simulink model "admire_sim_wal"  (Simulink 3.00)
settings: Solver=ode4  SolverMode=SingleTasking  StartTime=0.0  StopTime=7.5  FixedStep=0.01  RelTol=1e-3  AbsTol=1e-6
values from neighbouring files (symbols this model uses):
  x0 = [ max(eyp,zeros(n,1));max(-eyp,zeros(n,1));zeros(2*m,1)]    [LPwrap.m]
undefined symbols (not defined in the file or in its folder): dalpha_err, dalt_err, dbeta_err, dCl_beta, dCl_dai, dCl_day, dCl_dr, dCl_p, dCl_r, dCm_alpha, dCm_dei, dCm_dey, dCm_dne, dCm_q, dCn_beta, dCn_dna, dCn_dr, dCn_p, dCn_r, dCn_zero, ddc_bw, ddc_rate, ddei_bw, ddei_rate, ddey_bw, ddey_rate, ddle_bw, ddle_rate, ddr_bw, ddr_rate, dIxx, dIxz, dIyy, dIzz, dmass, dVt_err, dxcg, dycg, dzcg, rlimit_c, rlimit_ie, rlimit_le, rlimit_oe, rlimit_r, u0corr, u0fcs, u0new, x0diff, y0bare
libraries: simulink_extras x27, simulink3 x22
(part 1 of 2)
settings Model: RTWOptions="-aLogVarNameModifier=\"rt_\" -aExtMode=0 -aRollThreshold=5 -aShowEliminatedStatements=1 -aRTWVerbose=1 -aInlineInvariantSignals=1 -aLocalBlockOutputs=1 -aInlineParameters=0"  RTWTemplateMakefile=grt_adm5p3.tmf  LastModifiedBy=hkg  ModifiedComment=nnt -- Mon Jun 05 13:08:11 2000 -- Version 3.42
settings Model: ModifiedHistory=|
  | nnt -- Mon Jun 05 13:08:11 2000 -- Version 3.42
  | 
  | 
  | nnt -- Mon Jun 05 11:01:33 2000 -- Version 3.41
  | 
  | 
  | nnt -- Mon Jun 05 10:57:40 2000 -- Version 3.40
  | 
  | 
  | nnt -- Mon Jun 05 10:56:46 2000 -- Version 3.39
  | 
  | 
  | hkg -- Thu Apr 13 16:38:30 2000 -- Version 3.38
  | Bug fix: all rate limiters were set with the canard parameters, now they get individual settings..
  | 
  | hkg -- Thu Apr 13 10:24:31 2000 -- Version 3.37
  | Inserted 3.0 version number in Level 1, changed month to April.
  | 
  | hkg -- Tue Apr 11 10:36:55 2000 -- Version 3.36
  | dtz re-connected
  | 
  | hkg -- Tue Apr 11 10:28:52 2000 -- Version 3.35
  | Changed the roll force saturation to +-80 N
  | 
  | hkg -- Tue Apr 11 09:23:02 2000 -- Version 3.34
  | All signal generators on Level 1 are now set to sine wave
  | 
  | hkg -- Mon Apr 10 15:03:16 2000 -- Version 3.33
  | New names for the RL_choice blocks
  | 
  | fosimadmin -- Mon Apr 10 13:44:14 2000 -- Version 3.32
  | Hkg actually. Nothing special
  | 
  | hkg -- Fri Apr 07 14:32:16 2000 -- Version 3.31
  | A few corrections to the names
  | 
  | hkg -- Fri Apr 07 14:16:55 2000 -- Version 3.30
  | Added unique names inside Saab and DASA rate limiters for left elevons, rudder and
  | leading-edge flaps.
  | hkg -- Fri Apr 07 14:04:35 2000 -- Version 3.29
  | Added unique names inside SAAB and DASA rate limiters for canard and right outer and
  | inner elevons.
  | hkg -- Thu Apr 06 17:23:24 2000 -- Version 3.28
  | Inserted unique names for rate limiters and multiport switches in the rate limiter selection blocks.
  | hkg -- Thu Apr 06 16:09:22 2000 -- Version 3.27
  | Disconnected dtz again. Chosen grt_adm5p3.tmf as template makefile. Code generation seems to work.
  | hyd -- Tue Mar 28 15:20:39 2000 -- Version 3.26
  | hyd -- Tue Mar 28 14:28:32 2000 -- Version 3.25
  | hyd -- Tue Mar 28 11:30:24 2000 -- Version 3.24
  | hyd -- Mon Mar 27 15:22:27 2000 -- Version 3.23
  | hyd -- Mon Mar 27 13:42:12 2000 -- Version 3.22
  | hyd -- Mon Mar 27 10:51:54 2000 -- Version 3.21
  | hyd -- Fri Mar 24 13:18:05 2000 -- Version 3.20
  | hyd -- Fri Mar 24 12:50:02 2000 -- Version 3.19
  | hyd -- Fri Mar 24 11:54:23 2000 -- Version 3.18
  | hyd -- Thu Mar 23 15:20:42 2000 -- Version 3.17
  | hyd -- Thu Mar 23 15:17:54 2000 -- Version 3.16
  | hyd -- Wed Mar 22 09:38:49 2000 -- Version 3.15
  | hyd -- Tue Mar 21 14:06:08 2000 -- Version 3.14
  | hyd -- Mon Mar 20 14:42:54 2000 -- Version 3.13
  | hyd -- Wed Mar 15 13:37:48 2000 -- Version 3.12
  | hyd -- Wed Mar 15 12:35:54 2000 -- Version 3.11
  | jnr -- Tue Mar 14 16:36:26 2000 -- Version 3.10
  | jnr -- Tue Mar 14 14:13:39 2000 -- Version 3.9
  | jnr -- Tue Mar 14 14:13:23 2000 -- Version 3.8
  | jnr -- Tue Mar 14 10:09:15 2000 -- Version 3.7
  | jnr -- Tue Mar 14 09:37:34 2000 -- Version 3.6
  | jnr -- Tue Mar 14 09:30:20 2000 -- Version 3.5
  | Add:
  | *proper stick gradients.
  | *correct gains for nz-control according to Åke Hydén.
  | *what transition region between q-control and nz-control is proper??
  | fll -- Fri Mar 03 09:53:48 2000 -- Version 3.4
  | changed name of "dtx" to "dty" (horizontal nozzle deflection)
  | fll -- Thu Mar 02 12:51:23 2000 -- Version 3.3
  | Reducesed the number of integrators to one in the longitudinal controller.
  | fll -- Thu Mar 02 12:30:52 2000 -- Version 3.2
  | Moved the blending function in the Nz and q controller.
  | fll -- Thu Mar 02 10:50:25 2000 -- Version 3.1
  | Changed input blocks to "Signal generator"
  | fll -- Thu Mar 02 10:50:25 2000 -- Version 3.0
  | Version 3.0 is modified according to comments from users

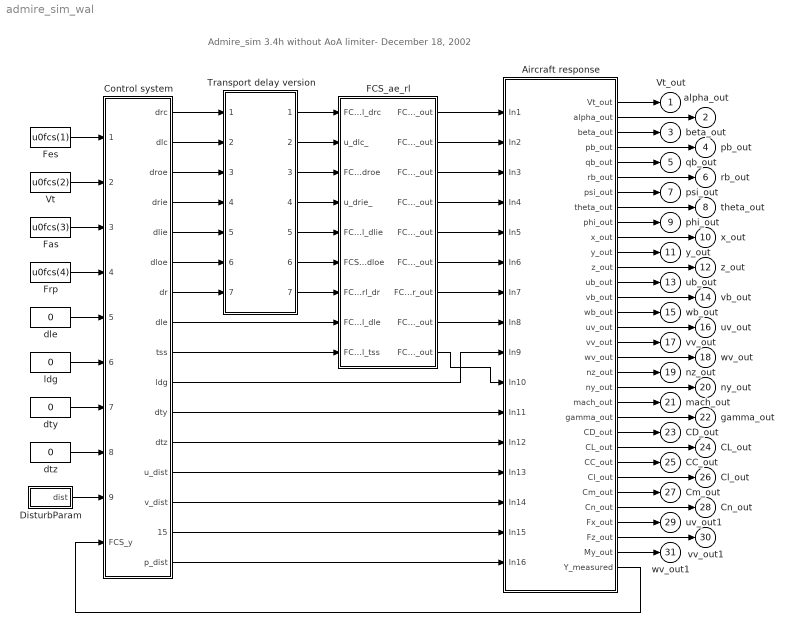
== system admire_sim_wal ==
  note: Admire_sim 3.4h without AoA limiter- December 18, 2002
  Aircraft response : Subsystem
      mask Display: disp('Aircraft\nResponse')
  Control system : Subsystem
      mask Display: disp('Control\nSystem')
  DisturbParam : Subsystem
  FCS_ae_rl : Subsystem
      mask Display: disp('Saturators\nRatelimiters\nand\nActuators')
  Fas : Constant  Value=u0fcs(3)
  Fes : Constant  Value=u0fcs(1)
  Frp : Constant  Value=u0fcs(4)
  Transport delay version : Subsystem
      mask Display: disp('Total\nComputer\nDelay\n\nTransport\ndelay\nversion')
  Vt : Constant  Value=u0fcs(2)
  dle : Constant  Value=0
  dty : Constant  Value=0
  dtz : Constant  Value=0
  ldg : Constant  Value=0
  Vt_out : Outport  Port=1  InitialOutput=0
  alpha_out : Outport  Port=2  InitialOutput=0
  beta_out : Outport  Port=3  InitialOutput=0
  pb_out : Outport  Port=4  InitialOutput=0
  qb_out : Outport  Port=5  InitialOutput=0
  rb_out : Outport  Port=6  InitialOutput=0
  psi_out : Outport  Port=7  InitialOutput=0
  theta_out : Outport  Port=8  InitialOutput=0
  phi_out : Outport  Port=9  InitialOutput=0
  x_out : Outport  Port=10  InitialOutput=0
  y_out : Outport  Port=11  InitialOutput=0
  z_out : Outport  Port=12  InitialOutput=0
  ub_out : Outport  Port=13  InitialOutput=0
  vb_out : Outport  Port=14  InitialOutput=0
  wb_out : Outport  Port=15  InitialOutput=0
  uv_out : Outport  Port=16  InitialOutput=0
  vv_out : Outport  Port=17  InitialOutput=0
  wv_out : Outport  Port=18  InitialOutput=0
  nz_out : Outport  Port=19  InitialOutput=0
  ny_out : Outport  Port=20  InitialOutput=0
  mach_out : Outport  Port=21  InitialOutput=0
  gamma_out : Outport  Port=22  InitialOutput=0
  CD_out : Outport  Port=23  InitialOutput=0
  CL_out : Outport  Port=24  InitialOutput=0
  CC_out : Outport  Port=25  InitialOutput=0
  Cl_out : Outport  Port=26  InitialOutput=0
  Cm_out : Outport  Port=27  InitialOutput=0
  Cn_out : Outport  Port=28  InitialOutput=0
  uv_out1 : Outport  Port=29  InitialOutput=0
  vv_out1 : Outport  Port=30  InitialOutput=0
  wv_out1 : Outport  Port=31  InitialOutput=0
  wires:
  Aircraft response/1(Vt_out) -> Vt_out/1
  Aircraft response/3(beta_out) -> beta_out/1
  Aircraft response/5(qb_out) -> qb_out/1
  Aircraft response/7(psi_out) -> psi_out/1
  Aircraft response/9(phi_out) -> phi_out/1
  Aircraft response/11(y_out) -> y_out/1
  Aircraft response/13(ub_out) -> ub_out/1
  Aircraft response/15(wb_out) -> wb_out/1
  Aircraft response/19(nz_out) -> nz_out/1
  FCS_ae_rl/8(FCS_ae_rl_dle_out) -> Aircraft response/8(In8)
  FCS_ae_rl/7(FCS_ae_rl_dr_out) -> Aircraft response/7(In7)
  FCS_ae_rl/6(FCS_ae_rl_dloe_out) -> Aircraft response/6(In6)
  FCS_ae_rl/5(FCS_ae_rl_dlie_out) -> Aircraft response/5(In5)
  FCS_ae_rl/4(FCS_ae_rl_drie_out) -> Aircraft response/4(In4)
  FCS_ae_rl/3(FCS_ae_rl_droe_out) -> Aircraft response/3(In3)
  FCS_ae_rl/2(FCS_ae_rl_dlc_out) -> Aircraft response/2(In2)
  FCS_ae_rl/1(FCS_ae_rl_drc_out) -> Aircraft response/1(In1)
  FCS_ae_rl/9(FCS_ae_rl_tss_out) -> Aircraft response/10(In10)
  Transport delay version/1(FCS_ae_rl_del_drc_delayed) -> FCS_ae_rl/1(FCS_ae_rl_drc)
  Transport delay version/2(FCS_ae_rl_del_dlc_delayed) -> FCS_ae_rl/2(u_dlc_)
  Transport delay version/3(FCS_ae_rl_del_droe_delayed) -> FCS_ae_rl/3(FCS_ae_rl_droe)
  Transport delay version/4(FCS_ae_rl_del_drie_delayed) -> FCS_ae_rl/4(u_drie_)
  Transport delay version/5(FCS_ae_rl_del_dlie_delayed) -> FCS_ae_rl/5(FCS_ae_rl_dlie)
  Transport delay version/6(FCS_ae_rl_del_dloe_delayed) -> FCS_ae_rl/6(FCS_ae_rl_dloe)
  Transport delay version/7(FCS_ae_rl_del_dr_delayed) -> FCS_ae_rl/7(FCS_ae_rl_dr)
  Aircraft response/17(vv_out) -> vv_out/1
  Aircraft response/21(mach_out) -> mach_out/1
  Aircraft response/23(CD_out) -> CD_out/1
  Aircraft response/25(CC_out) -> CC_out/1
  Aircraft response/27(Cm_out) -> Cm_out/1
  Aircraft response/29(Fx_out) -> uv_out1/1
  Aircraft response/31(My_out) -> wv_out1/1
  Aircraft response/2(alpha_out) -> alpha_out/1
  Aircraft response/22(gamma_out) -> gamma_out/1
  Aircraft response/4(pb_out) -> pb_out/1
  Aircraft response/6(rb_out) -> rb_out/1
  Aircraft response/8(theta_out) -> theta_out/1
  Aircraft response/10(x_out) -> x_out/1
  Aircraft response/14(vb_out) -> vb_out/1
  Aircraft response/16(uv_out) -> uv_out/1
  Aircraft response/18(wv_out) -> wv_out/1
  Aircraft response/20(ny_out) -> ny_out/1
  Aircraft response/12(z_out) -> z_out/1
  Aircraft response/24(CL_out) -> CL_out/1
  Aircraft response/26(Cl_out) -> Cl_out/1
  Aircraft response/28(Cn_out) -> Cn_out/1
  Aircraft response/30(Fz_out) -> vv_out1/1
  Control system/1(drc) -> Transport delay version/1(FCS_ae_rl_del_drc)
  Control system/2(dlc) -> Transport delay version/2(FCS_ae_rl_del_dlc)
  Control system/3(droe) -> Transport delay version/3(FCS_ae_rl_del_droe)
  Control system/4(drie) -> Transport delay version/4(FCS_ae_rl_del_drie)
  Control system/5(dlie) -> Transport delay version/5(FCS_ae_rl_del_dlie)
  Control system/6(dloe) -> Transport delay version/6(FCS_ae_rl_del_dloe)
  Control system/7(dr) -> Transport delay version/7(FCS_ae_rl_del_dr)
  Control system/8(dle) -> FCS_ae_rl/8(FCS_ae_rl_dle)
  Control system/9(tss) -> FCS_ae_rl/9(FCS_ae_rl_tss)
  Control system/10(ldg) -> Aircraft response/9(In9)
  Control system/11(dty) -> Aircraft response/11(In11)
  Control system/13(u_dist) -> Aircraft response/13(In13)
  Control system/14(v_dist) -> Aircraft response/14(In14)
  Control system/15(w_dist) -> Aircraft response/15(In15)
  Control system/16(p_dist) -> Aircraft response/16(In16)
  DisturbParam/1(dist) -> Control system/9(FCS_dist)
  dtz/1 -> Control system/8(FCS_dtz)
  dty/1 -> Control system/7(FCS_dty)
  ldg/1 -> Control system/6(FCS_ldg)
  dle/1 -> Control system/5(FCS_dle)
  Frp/1 -> Control system/4(FCS_Frp)
  Aircraft response/32(Y_measured) -> Control system/10(FCS_y)
  Control system/12(dtz) -> Aircraft response/12(In12)
  Fas/1 -> Control system/3(FCS_Fas)
  Vt/1 -> Control system/2(FCS_Vt)
  Fes/1 -> Control system/1(FCS_Fes)

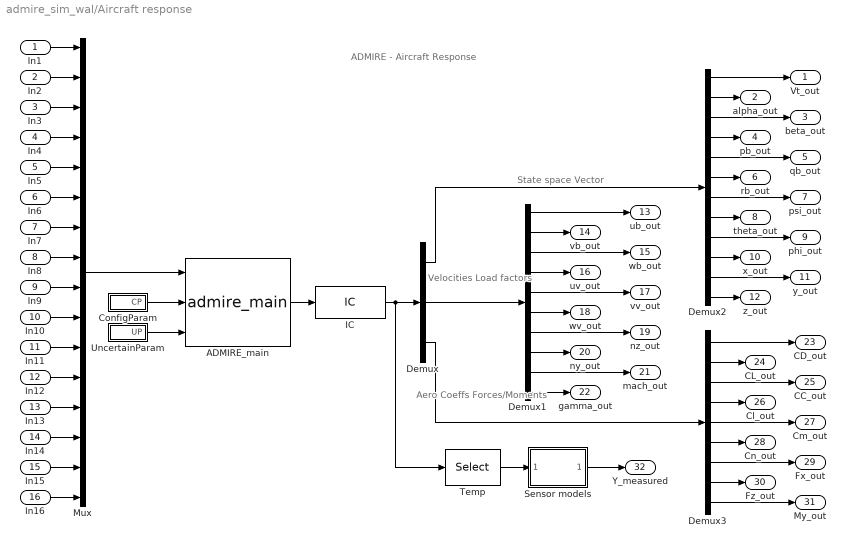
== system admire_sim_wal/Aircraft response ==
  note: State space Vector
  note: Velocities
      | Load factors
  note: Aero Coeffs
      | Forces/Moments
  note: ADMIRE - Aircraft Response
  In1 : Inport  Port=1  PortWidth=-1  SampleTime=-1  DataType=auto
      settings: SignalType=auto
  In2 : Inport  Port=2  PortWidth=-1  SampleTime=-1  DataType=auto
      settings: SignalType=auto
  In3 : Inport  Port=3  PortWidth=-1  SampleTime=-1  DataType=auto
      settings: SignalType=auto
  In4 : Inport  Port=4  PortWidth=-1  SampleTime=-1  DataType=auto
      settings: SignalType=auto
  In5 : Inport  Port=5  PortWidth=-1  SampleTime=-1  DataType=auto
      settings: SignalType=auto
  In6 : Inport  Port=6  PortWidth=-1  SampleTime=-1  DataType=auto
      settings: SignalType=auto
  In7 : Inport  Port=7  PortWidth=-1  SampleTime=-1  DataType=auto
      settings: SignalType=auto
  In8 : Inport  Port=8  PortWidth=-1  SampleTime=-1  DataType=auto
      settings: SignalType=auto
  In9 : Inport  Port=9  PortWidth=-1  SampleTime=-1  DataType=auto
      settings: SignalType=auto
  In10 : Inport  Port=10  PortWidth=-1  SampleTime=-1  DataType=auto
      settings: SignalType=auto
  In11 : Inport  Port=11  PortWidth=-1  SampleTime=-1  DataType=auto
      settings: SignalType=auto
  In12 : Inport  Port=12  PortWidth=-1  SampleTime=-1  DataType=auto
      settings: SignalType=auto
  In13 : Inport  Port=13  PortWidth=-1  SampleTime=-1  DataType=auto
      settings: SignalType=auto
  In14 : Inport  Port=14  PortWidth=-1  SampleTime=-1  DataType=auto
      settings: SignalType=auto
  In15 : Inport  Port=15  PortWidth=-1  SampleTime=-1  DataType=auto
      settings: SignalType=auto
  In16 : Inport  Port=16  PortWidth=-1  SampleTime=-1  DataType=auto
      settings: SignalType=auto
  ADMIRE_main : S-Function  FunctionName=admire_main  Parameters=x0bare dx0bare  PortCounts=[]  SFunctionModules=''
      mask Type: ADMIRE C-code block
      mask Description:
      | Main block describing the ADMIRE.
      | To use HELP, start any Internet browser.
      mask Help:
      | The aircraft it self is a C-code file that calculates the dynamics of the structure and the air surrounding it.<br>
      | The simulation requires an initial vector of values called x0 containing the following variables.<br><br>
      | 
      | Vt_init     --     initial airspeed.                        [m/s]<br>
      | alpha_init --    initial angle of attack.             [rad]<br>
      | beta_init    --   initial angle of sideslip.            [rad]<br>
      | pb_init     --     initial roll angular rate.             [rad/s]<br>
      | qb_init     --     initial pitch angular rate.          [rad/s]<br>
      | rb_init       --    initial yaw angular rate.           [rad/s]<br>
      | psi_init      --    initial euler angles (azimuth)    [rad]<br>
      | theta_init   --   initial (elevation)                      [rad]<br>
      | phi_init      --   initial (bank)                             [rad]<br>
      | xv_init      --    initial x position in Fv                [m]<br>
      | yv_init        --  initial y                                     [m]<br>
      | zv_init       --   initial z                                     [m]<br>
      mask Display:
      | plot([18 12 3 2 2 8 11],[7 4 1 1 2 8 11])
      | plot([13 11 13 15 15 13],[12 11 16 17 13 12])
      | plot([15 17 20 23 30 17],[13 14 24 25 20 14])
      | plot([30 38 40 38 30],[19 31 32 22 19])
      | plot([38.5 41 36 22 41 43 36],[23 21 16 10 8 10 16])
      | plot([15 19 25 24 15],[7 9 9 8 7])
      | plot([8 11 13 14 9 8],[8 11 12 10 7 8])
      | plot([21 23],[9 10])
      | plot([30 31],[20 20.5])
  ConfigParam : Subsystem
  Demux : Demux  Outputs=[12 10 9]
  Demux1 : Demux  Outputs=10
  Demux2 : Demux  Outputs=12
  Demux3 : Demux  Outputs=9
  IC : InitialCondition  Value=y0bare(1:31)
  Mux : Mux  Inputs=16
      settings: DisplayOption=none
  Sensor models : Subsystem
      mask Display: disp('Sensors')
  Temp : Selector  Elements=[1:28]  InputPortWidth=31
  UncertainParam : Subsystem
      mask Display: plot([0 10 5 0],[0 0 8.6603 0])
  Vt_out : Outport  Port=1
  alpha_out : Outport  Port=2
  beta_out : Outport  Port=3
  pb_out : Outport  Port=4
  qb_out : Outport  Port=5
  rb_out : Outport  Port=6
  psi_out : Outport  Port=7
  theta_out : Outport  Port=8
  phi_out : Outport  Port=9
  x_out : Outport  Port=10
  y_out : Outport  Port=11
  z_out : Outport  Port=12
  ub_out : Outport  Port=13
  vb_out : Outport  Port=14
  wb_out : Outport  Port=15
  uv_out : Outport  Port=16
  vv_out : Outport  Port=17
  wv_out : Outport  Port=18
  nz_out : Outport  Port=19
  ny_out : Outport  Port=20
  mach_out : Outport  Port=21
  gamma_out : Outport  Port=22
  CD_out : Outport  Port=23
  CL_out : Outport  Port=24
  CC_out : Outport  Port=25
  Cl_out : Outport  Port=26
  Cm_out : Outport  Port=27
  Cn_out : Outport  Port=28
  Fx_out : Outport  Port=29
  Fz_out : Outport  Port=30
  My_out : Outport  Port=31
  Y_measured : Outport  Port=32
  wires:
  Mux/1 -> ADMIRE_main/1
  In15/1 -> Mux/15
  In16/1 -> Mux/16
  In1/1 -> Mux/1
  In2/1 -> Mux/2
  In3/1 -> Mux/3
  In4/1 -> Mux/4
  In5/1 -> Mux/5
  In6/1 -> Mux/6
  In7/1 -> Mux/7
  In8/1 -> Mux/8
  In9/1 -> Mux/9
  In10/1 -> Mux/10
  In11/1 -> Mux/11
  In12/1 -> Mux/12
  In13/1 -> Mux/13
  In14/1 -> Mux/14
  Demux/2 -> Demux1/1
  Demux/1 -> Demux2/1
  Demux/3 -> Demux3/1
  Demux3/2 -> CL_out/1
  Demux3/4 -> Cl_out/1
  Demux3/6 -> Cn_out/1
  Demux3/8 -> Fz_out/1
  Demux3/1 -> CD_out/1
  Demux3/3 -> CC_out/1
  Demux3/5 -> Cm_out/1
  Demux3/7 -> Fx_out/1
  Demux3/9 -> My_out/1
  Demux2/2 -> alpha_out/1
  Demux2/4 -> pb_out/1
  Demux2/6 -> rb_out/1
  Demux2/8 -> theta_out/1
  Demux2/10 -> x_out/1
  Demux2/12 -> z_out/1
  Demux2/1 -> Vt_out/1
  Demux2/3 -> beta_out/1
  Demux2/5 -> qb_out/1
  Demux2/7 -> psi_out/1
  Demux2/9 -> phi_out/1
  Demux2/11 -> y_out/1
  Demux1/2 -> vb_out/1
  Demux1/4 -> uv_out/1
  Demux1/6 -> wv_out/1
  Demux1/8 -> ny_out/1
  Demux1/10 -> gamma_out/1
  Demux1/1 -> ub_out/1
  Demux1/3 -> wb_out/1
  Demux1/5 -> vv_out/1
  Demux1/7 -> nz_out/1
  Demux1/9 -> mach_out/1
  Sensor models/1(admire_sensed_out) -> Y_measured/1
  Temp/1 -> Sensor models/1(admire_out)
  ConfigParam/1(CP) -> ADMIRE_main/2
  UncertainParam/1(UP) -> ADMIRE_main/3
  ADMIRE_main/1 -> IC/1
  IC/1 -> Demux/1, Temp/1

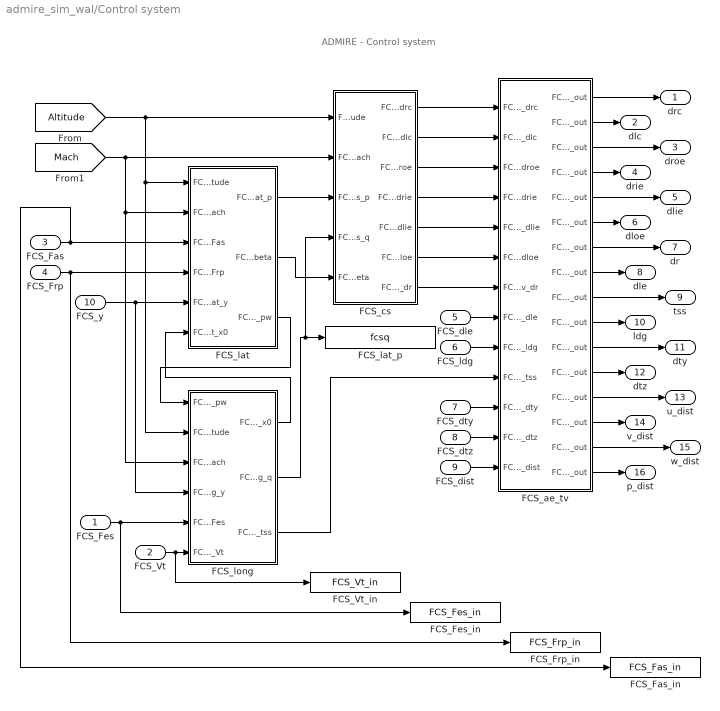
== system admire_sim_wal/Control system ==
  note: ADMIRE - Control system
  FCS_Fes : Inport  Port=1  PortWidth=-1  SampleTime=-1  DataType=auto
      settings: SignalType=auto
  FCS_Vt : Inport  Port=2  PortWidth=-1  SampleTime=-1  DataType=auto
      settings: SignalType=auto
  FCS_Fas : Inport  Port=3  PortWidth=-1  SampleTime=-1  DataType=auto
      settings: SignalType=auto
  FCS_Frp : Inport  Port=4  PortWidth=-1  SampleTime=-1  DataType=auto
      settings: SignalType=auto
  FCS_dle : Inport  Port=5  PortWidth=-1  SampleTime=-1  DataType=auto
      settings: SignalType=auto
  FCS_ldg : Inport  Port=6  PortWidth=-1  SampleTime=-1  DataType=auto
      settings: SignalType=auto
  FCS_dty : Inport  Port=7  PortWidth=-1  SampleTime=-1  DataType=auto
      settings: SignalType=auto
  FCS_dtz : Inport  Port=8  PortWidth=-1  SampleTime=-1  DataType=auto
      settings: SignalType=auto
  FCS_dist : Inport  Port=9  PortWidth=-1  SampleTime=-1  DataType=auto
      settings: SignalType=auto
  FCS_y : Inport  Port=10  PortWidth=-1  SampleTime=-1  DataType=auto
      settings: SignalType=auto
  FCS_Fas_in : ToWorkspace  VariableName=FCS_Fas_in  SampleTime=-1  SaveFormat=Matrix
  FCS_Fes_in : ToWorkspace  VariableName=FCS_Fes_in  SampleTime=-1  SaveFormat=Matrix
  FCS_Frp_in : ToWorkspace  VariableName=FCS_Frp_in  SampleTime=-1  SaveFormat=Matrix
  FCS_Vt_in : ToWorkspace  VariableName=FCS_Vt_in  SampleTime=-1  SaveFormat=Matrix
  FCS_ae_tv : Subsystem
      mask Display: disp('Adding\ntrim\nvalues')
  "FCS_cs " : Subsystem
      mask Display: disp('FCS_cs')
  FCS_lat : Subsystem
      mask Display: disp('FCS_lat')
  FCS_lat_p : ToWorkspace  VariableName=fcsq  SampleTime=-1  SaveFormat=Matrix
  FCS_long : Subsystem
      mask Display: disp('FCS_long')
  drc : Outport  Port=1
  dlc : Outport  Port=2
  droe : Outport  Port=3
  drie : Outport  Port=4
  dlie : Outport  Port=5
  dloe : Outport  Port=6
  dr : Outport  Port=7
  dle : Outport  Port=8
  tss : Outport  Port=9
  ldg : Outport  Port=10
  dty : Outport  Port=11
  dtz : Outport  Port=12
  u_dist : Outport  Port=13
  v_dist : Outport  Port=14
  w_dist : Outport  Port=15
  p_dist : Outport  Port=16
  wires:
  FCS_long/1(FCS_long_x0) -> FCS_lat/6(FCS_lat_x0)
  FCS_lat/3(FCS_lat_pw) -> FCS_long/1("FCS_long_pw ")
  FCS_lat/2("FCS_lat_beta ") -> "FCS_cs "/5(FCS_cs_beta)
  FCS_lat/1("FCS_lat_p ") -> "FCS_cs "/3(FCS_cs_p)
  "FCS_cs "/1(FCS_cs_drc) -> FCS_ae_tv/1(FCS_ae_tv_drc)
  "FCS_cs "/2(FCS_cs_dlc) -> FCS_ae_tv/2(FCS_ae_tv_dlc)
  "FCS_cs "/3(FCS_cs_droe) -> FCS_ae_tv/3(FCS_ae_tv_droe)
  "FCS_cs "/4(FCS_cs_drie) -> FCS_ae_tv/4(FCS_ae_tv_drie)
  "FCS_cs "/5(FCS_cs_dlie) -> FCS_ae_tv/5(FCS_ae_tv_dlie)
  "FCS_cs "/6(FCS_cs_dloe) -> FCS_ae_tv/6(FCS_ae_tv_dloe)
  "FCS_cs "/7(FCS_cs_dr) -> FCS_ae_tv/7(FCS_ae_tv_dr)
  FCS_ae_tv/1("FCS_ae_tv_drc_out ") -> drc/1
  FCS_ae_tv/2("FCS_ae_tv_dlc_out ") -> dlc/1
  FCS_ae_tv/3("FCS_ae_tv_droe_out ") -> droe/1
  FCS_ae_tv/4("FCS_ae_tv_drie_out ") -> drie/1
  FCS_ae_tv/5("FCS_ae_tv_dlie_out ") -> dlie/1
  FCS_ae_tv/6("FCS_ae_tv_dloe_out ") -> dloe/1
  FCS_ae_tv/7(FCS_ae_tv_dr _out) -> dr/1
  FCS_ae_tv/8("FCS_ae_tv_dle_out ") -> dle/1
  FCS_ae_tv/9("FCS_ae_tv_tss_out ") -> tss/1
  FCS_dle/1 -> FCS_ae_tv/8(FCS_ae_tv_dle)
  FCS_ae_tv/10("FCS_ae_tv_ldg_out ") -> ldg/1
  FCS_ldg/1 -> FCS_ae_tv/9(FCS_ae_tv_ldg)
  FCS_ae_tv/11(FCS_ae_tv_dty_out) -> dty/1
  FCS_ae_tv/12("FCS_ae_tv_dtz_out ") -> dtz/1
  FCS_ae_tv/13("FCS_ae_tv_u_dist_out ") -> u_dist/1
  FCS_dty/1 -> FCS_ae_tv/11(FCS_ae_tv_dty)
  FCS_ae_tv/14("FCS_ae_tv_v_dist_out ") -> v_dist/1
  FCS_dtz/1 -> FCS_ae_tv/12(FCS_ae_tv_dtz)
  FCS_ae_tv/15(FCS_ae_tv_w_dist _out) -> w_dist/1
  FCS_dist/1 -> FCS_ae_tv/13(FCS_ae_tv_dist)
  FCS_ae_tv/16("FCS_ae_tv_p_dist_out ") -> p_dist/1
  FCS_long/3(FCS_long_tss) -> FCS_ae_tv/10(FCS_ae_tv_tss)
  [Mach] -> "FCS_cs "/2(FCS_cs_Mach), FCS_lat/2("FCS_lat_Mach "), FCS_long/3(FCS_long_Mach)
  [Altitude] -> "FCS_cs "/1(FCS_cs_Altitude), FCS_lat/1("FCS_lat_Altitude "), FCS_long/2("FCS_long_Altitude ")
  FCS_y/1 -> FCS_lat/5("FCS_lat_y "), FCS_long/4(FCS_long_y)
  FCS_Vt/1 -> FCS_long/6("FCS_long_Vt "), FCS_Vt_in/1
  FCS_Fes/1 -> FCS_long/5(FCS_long_Fes), FCS_Fes_in/1
  FCS_Frp/1 -> FCS_lat/4(FCS_lat_Frp), FCS_Frp_in/1
  FCS_Fas/1 -> FCS_lat/3(FCS_lat_Fas), FCS_Fas_in/1
  FCS_long/2(FCS_long_q) -> FCS_lat_p/1, "FCS_cs "/4(FCS_cs_q)

== system admire_sim_wal/DisturbParam ==
  note: Level II
  Mux : Mux  Inputs=4
      settings: DisplayOption=none
  "p_dist " : Constant  Value=0
  "u_dist " : Constant  Value=0
  "v_dist " : Constant  Value=0
  "w_dist " : Constant  Value=0
  dist : Outport  Port=1
  wires:
  "p_dist "/1 -> Mux/4
  "w_dist "/1 -> Mux/3
  "v_dist "/1 -> Mux/2
  "u_dist "/1 -> Mux/1
  Mux/1 -> dist/1

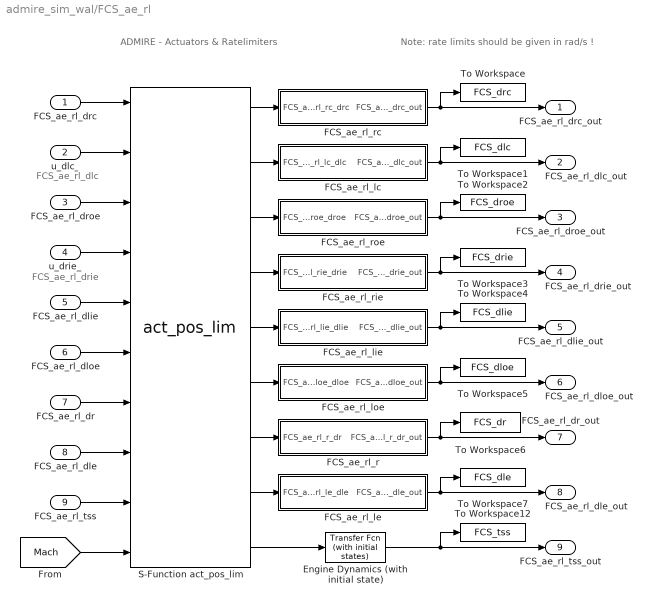
== system admire_sim_wal/FCS_ae_rl ==
  note: Note: rate limits should be given
      | in rad/s !
  note: FCS_ae_rl_dlc
  note: FCS_ae_rl_drie
  note: ADMIRE - Actuators & Ratelimiters
  FCS_ae_rl_drc : Inport  Port=1  PortWidth=-1  SampleTime=-1  DataType=auto
      settings: SignalType=auto
  u_dlc_ : Inport  Port=2  PortWidth=-1  SampleTime=-1  DataType=auto
      settings: SignalType=auto
  FCS_ae_rl_droe : Inport  Port=3  PortWidth=-1  SampleTime=-1  DataType=auto
      settings: SignalType=auto
  u_drie_ : Inport  Port=4  PortWidth=-1  SampleTime=-1  DataType=auto
      settings: SignalType=auto
  FCS_ae_rl_dlie : Inport  Port=5  PortWidth=-1  SampleTime=-1  DataType=auto
      settings: SignalType=auto
  FCS_ae_rl_dloe : Inport  Port=6  PortWidth=-1  SampleTime=-1  DataType=auto
      settings: SignalType=auto
  FCS_ae_rl_dr : Inport  Port=7  PortWidth=-1  SampleTime=-1  DataType=auto
      settings: SignalType=auto
  FCS_ae_rl_dle : Inport  Port=8  PortWidth=-1  SampleTime=-1  DataType=auto
      settings: SignalType=auto
  FCS_ae_rl_tss : Inport  Port=9  PortWidth=-1  SampleTime=-1  DataType=auto
      settings: SignalType=auto
  Engine Dynamics (with initial state) : simulink_extras/Additional Linear/Transfer Fcn (with initial states)  N=[1]  D="[2  1]"  X0=x0(9)
  FCS_ae_rl_lc : Subsystem
      mask Display: disp(' Ratelimiter and Dynamics\nServo: lc')
  FCS_ae_rl_le : Subsystem
      mask Display: disp(' Ratelimiter and Dynamics\nServo: le')
  FCS_ae_rl_lie : Subsystem
      mask Display: disp(' Ratelimiter and Dynamics\nServo: lie')
  FCS_ae_rl_loe : Subsystem
      mask Display: disp(' Ratelimiter and Dynamics\nServo: loe')
  FCS_ae_rl_r : Subsystem
      mask Display: disp(' Ratelimiter and Dynamics\nServo: r')
  FCS_ae_rl_rc : Subsystem
      mask Display: disp(' Ratelimiter and Dynamics\nServo: rc')
  FCS_ae_rl_rie : Subsystem
      mask Display: disp(' Ratelimiter and Dynamics\nServo: rie')
  FCS_ae_rl_roe : Subsystem
      mask Display: disp(' Ratelimiter and Dynamics\nServo: roe')
  S-Function act_pos_lim : S-Function  FunctionName=act_pos_lim  PortCounts=[]  SFunctionModules=''
      mask Display:
      | plot([-30 30],[-30 30])
      | plot([0 0],[-30 30])
      | plot([-50 50],[0 0])
      | plot([30 50],[30 30])
      | plot([-50 -30],[-30 -30])
      | plot([-5 0],[25 30])
      | plot([5 0],[25 30])
      | plot([45 50],[3 0])
      | plot([45 50],[-3 0])
      | text(-21,26,'out')
      | text(30,-2,'in')
  To Workspace : ToWorkspace  VariableName=FCS_drc  SampleTime=-1  SaveFormat=Matrix
  To Workspace1 : ToWorkspace  VariableName=FCS_dlc  SampleTime=-1  SaveFormat=Matrix
  To Workspace12 : ToWorkspace  VariableName=FCS_tss  SampleTime=-1  SaveFormat=Matrix
  To Workspace2 : ToWorkspace  VariableName=FCS_droe  SampleTime=-1  SaveFormat=Matrix
  To Workspace3 : ToWorkspace  VariableName=FCS_drie  SampleTime=-1  SaveFormat=Matrix
  To Workspace4 : ToWorkspace  VariableName=FCS_dlie  SampleTime=-1  SaveFormat=Matrix
  To Workspace5 : ToWorkspace  VariableName=FCS_dloe  SampleTime=-1  SaveFormat=Matrix
  To Workspace6 : ToWorkspace  VariableName=FCS_dr  SampleTime=-1  SaveFormat=Matrix
  To Workspace7 : ToWorkspace  VariableName=FCS_dle  SampleTime=-1  SaveFormat=Matrix
  FCS_ae_rl_drc_out : Outport  Port=1
  FCS_ae_rl_dlc_out : Outport  Port=2
  FCS_ae_rl_droe_out : Outport  Port=3
  FCS_ae_rl_drie_out : Outport  Port=4
  FCS_ae_rl_dlie_out : Outport  Port=5
  FCS_ae_rl_dloe_out : Outport  Port=6
  FCS_ae_rl_dr_out : Outport  Port=7
  FCS_ae_rl_dle_out : Outport  Port=8
  FCS_ae_rl_tss_out : Outport  Port=9
  wires:
  S-Function act_pos_lim/2 -> FCS_ae_rl_lc/1(FCS_ae_rl_lc_dlc)
  S-Function act_pos_lim/3 -> FCS_ae_rl_roe/1(FCS_ae_rl_roe_droe)
  S-Function act_pos_lim/5 -> FCS_ae_rl_lie/1(FCS_ae_rl_lie_dlie)
  S-Function act_pos_lim/6 -> FCS_ae_rl_loe/1(FCS_ae_rl_loe_dloe)
  S-Function act_pos_lim/7 -> FCS_ae_rl_r/1(FCS_ae_rl_r_dr)
  S-Function act_pos_lim/8 -> FCS_ae_rl_le/1(FCS_ae_rl_le_dle)
  S-Function act_pos_lim/9 -> Engine Dynamics (with initial state)/1
  S-Function act_pos_lim/1 -> FCS_ae_rl_rc/1(FCS_ae_rl_rc_drc)
  S-Function act_pos_lim/4 -> FCS_ae_rl_rie/1(FCS_ae_rl_rie_drie)
  [Mach] -> S-Function act_pos_lim/10
  u_dlc_/1 -> S-Function act_pos_lim/2
  FCS_ae_rl_drc/1 -> S-Function act_pos_lim/1
  FCS_ae_rl_droe/1 -> S-Function act_pos_lim/3
  FCS_ae_rl_dlie/1 -> S-Function act_pos_lim/5
  FCS_ae_rl_dloe/1 -> S-Function act_pos_lim/6
  FCS_ae_rl_dr/1 -> S-Function act_pos_lim/7
  u_drie_/1 -> S-Function act_pos_lim/4
  FCS_ae_rl_dle/1 -> S-Function act_pos_lim/8
  FCS_ae_rl_tss/1 -> S-Function act_pos_lim/9
  FCS_ae_rl_rc/1(FCS_ae_rl_rc_drc_out) -> To Workspace/1, FCS_ae_rl_drc_out/1
  FCS_ae_rl_lc/1(FCS_ae_rl_lc_dlc_out) -> To Workspace1/1, FCS_ae_rl_dlc_out/1
  Engine Dynamics (with initial state)/1 -> To Workspace12/1, FCS_ae_rl_tss_out/1
  FCS_ae_rl_le/1(FCS_ae_rl_le_dle_out) -> To Workspace7/1, FCS_ae_rl_dle_out/1
  FCS_ae_rl_r/1(FCS_ae_rl_r_dr_out) -> To Workspace6/1, FCS_ae_rl_dr_out/1
  FCS_ae_rl_loe/1(FCS_ae_rl_loe_dloe_out) -> To Workspace5/1, FCS_ae_rl_dloe_out/1
  FCS_ae_rl_lie/1(FCS_ae_rl_lie_dlie_out) -> To Workspace4/1, FCS_ae_rl_dlie_out/1
  FCS_ae_rl_roe/1(FCS_ae_rl_roe_droe_out) -> To Workspace2/1, FCS_ae_rl_droe_out/1
  FCS_ae_rl_rie/1(FCS_ae_rl_rie_drie_out) -> To Workspace3/1, FCS_ae_rl_drie_out/1

== system admire_sim_wal/Transport delay version ==
  note: Level V
  FCS_ae_rl_del_drc : Inport  Port=1  PortWidth=-1  SampleTime=-1  DataType=auto
      settings: SignalType=auto
  FCS_ae_rl_del_dlc : Inport  Port=2  PortWidth=-1  SampleTime=-1  DataType=auto
      settings: SignalType=auto
  FCS_ae_rl_del_droe : Inport  Port=3  PortWidth=-1  SampleTime=-1  DataType=auto
      settings: SignalType=auto
  FCS_ae_rl_del_drie : Inport  Port=4  PortWidth=-1  SampleTime=-1  DataType=auto
      settings: SignalType=auto
  FCS_ae_rl_del_dlie : Inport  Port=5  PortWidth=-1  SampleTime=-1  DataType=auto
      settings: SignalType=auto
  FCS_ae_rl_del_dloe : Inport  Port=6  PortWidth=-1  SampleTime=-1  DataType=auto
      settings: SignalType=auto
  FCS_ae_rl_del_dr : Inport  Port=7  PortWidth=-1  SampleTime=-1  DataType=auto
      settings: SignalType=auto
  "20 ms Transport Delay, initial input from  u0new 1" : TransportDelay  DelayTime=0.02  InitialInput=u0new(1)  BufferSize=100
  "20 ms Transport Delay, initial input from  u0new 2" : TransportDelay  DelayTime=0.02  InitialInput=u0new(2)  BufferSize=100
  "20 ms Transport Delay, initial input from  u0new 3" : TransportDelay  DelayTime=0.02  InitialInput=u0new(3)  BufferSize=100
  "20 ms Transport Delay, initial input from  u0new 4" : TransportDelay  DelayTime=0.02  InitialInput=u0new(4)  BufferSize=100
  "20 ms Transport Delay, initial input from  u0new 5" : TransportDelay  DelayTime=0.02  InitialInput=u0new(5)  BufferSize=100
  "20 ms Transport Delay, initial input from  u0new 6" : TransportDelay  DelayTime=0.02  InitialInput=u0new(6)  BufferSize=100
  "20 ms Transport Delay, initial input from  u0new 7" : TransportDelay  DelayTime=0.02  InitialInput=u0new(7)  BufferSize=100
  FCS_ae_rl_del_drc_delayed : Outport  Port=1
  FCS_ae_rl_del_dlc_delayed : Outport  Port=2
  FCS_ae_rl_del_droe_delayed : Outport  Port=3
  FCS_ae_rl_del_drie_delayed : Outport  Port=4
  FCS_ae_rl_del_dlie_delayed : Outport  Port=5
  FCS_ae_rl_del_dloe_delayed : Outport  Port=6
  FCS_ae_rl_del_dr_delayed : Outport  Port=7
  wires:
  FCS_ae_rl_del_dloe/1 -> "20 ms Transport Delay, initial input from  u0new 6"/1
  "20 ms Transport Delay, initial input from  u0new 5"/1 -> FCS_ae_rl_del_dlie_delayed/1
  FCS_ae_rl_del_dlie/1 -> "20 ms Transport Delay, initial input from  u0new 5"/1
  FCS_ae_rl_del_drie/1 -> "20 ms Transport Delay, initial input from  u0new 4"/1
  "20 ms Transport Delay, initial input from  u0new 3"/1 -> FCS_ae_rl_del_droe_delayed/1
  FCS_ae_rl_del_droe/1 -> "20 ms Transport Delay, initial input from  u0new 3"/1
  "20 ms Transport Delay, initial input from  u0new 7"/1 -> FCS_ae_rl_del_dr_delayed/1
  "20 ms Transport Delay, initial input from  u0new 1"/1 -> FCS_ae_rl_del_drc_delayed/1
  FCS_ae_rl_del_drc/1 -> "20 ms Transport Delay, initial input from  u0new 1"/1
  "20 ms Transport Delay, initial input from  u0new 2"/1 -> FCS_ae_rl_del_dlc_delayed/1
  FCS_ae_rl_del_dlc/1 -> "20 ms Transport Delay, initial input from  u0new 2"/1
  "20 ms Transport Delay, initial input from  u0new 4"/1 -> FCS_ae_rl_del_drie_delayed/1
  "20 ms Transport Delay, initial input from  u0new 6"/1 -> FCS_ae_rl_del_dloe_delayed/1
  FCS_ae_rl_del_dr/1 -> "20 ms Transport Delay, initial input from  u0new 7"/1

== system admire_sim_wal/Aircraft response/ConfigParam ==
  note: Level II
  "Ix " : Constant  Value=21000
  "Ixz " : Constant  Value=2500
  "Iy " : Constant  Value=81000
  "Iz " : Constant  Value=101000
  Mux : Mux  Inputs=8
      settings: DisplayOption=none
  "mass " : Constant  Value=9100
  "xcg " : Constant  Value=0*5.20
  "ycg " : Constant  Value=0
  "zcg " : Constant  Value=-0.15
  CP : Outport  Port=1  InitialOutput=0
  wires:
  "mass "/1 -> Mux/1
  "xcg "/1 -> Mux/2
  "ycg "/1 -> Mux/3
  "zcg "/1 -> Mux/4
  "Ix "/1 -> Mux/5
  "Iy "/1 -> Mux/6
  "Iz "/1 -> Mux/7
  "Ixz "/1 -> Mux/8
  Mux/1 -> CP/1

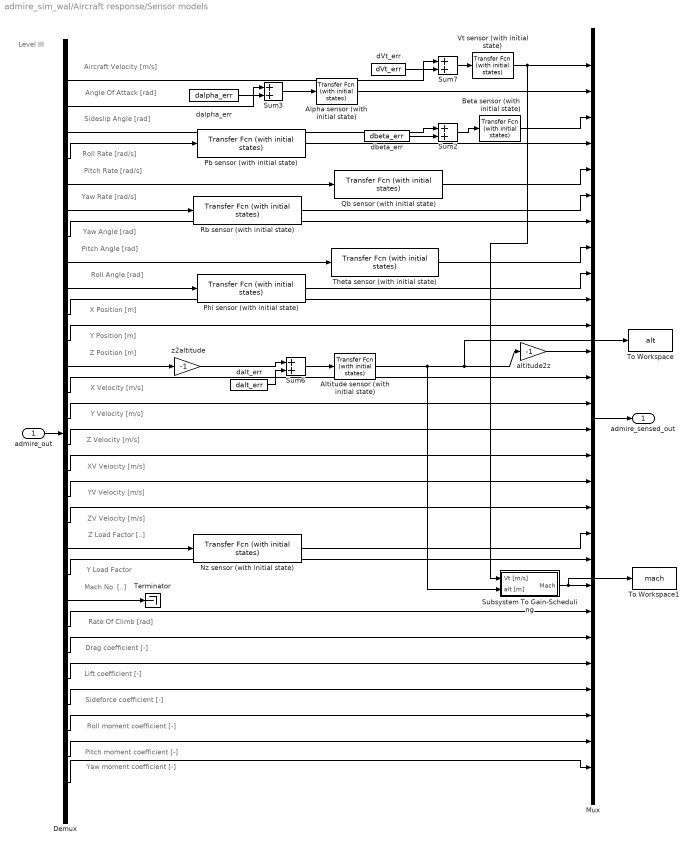
== system admire_sim_wal/Aircraft response/Sensor models ==
  note: Aircraft Velocity [m/s]
  note: Angle Of Attack [rad]
  note: Sideslip Angle [rad]
  note: Roll Rate [rad/s]
  note: Pitch Rate [rad/s]
  note: Yaw Rate [rad/s]
  note: Yaw Angle [rad]
  note: Pitch Angle [rad]
  note: Roll Angle [rad]
  note: X Position [m]
  note: Y Position [m]
  note: Z Position [m]
  note: X Velocity [m/s]
  note: Y Velocity [m/s]
  note: Z Velocity [m/s]
  note: ZV Velocity [m/s]
  note: YV Velocity [m/s]
  note: XV Velocity [m/s]
  note: Z Load Factor [..]
  note: Y Load Factor
  note: Mach No. [..]
  note: Rate Of Climb [rad]
  note: Drag coefficient [-]
  note: Lift coefficient [-]
  note: Sideforce coefficient [-]
  note: Roll moment coefficient [-]
  note: Pitch moment coefficient [-]
  note: Yaw moment coefficient [-]
  note: Level III
  admire_out : Inport  Port=1  PortWidth=-1  SampleTime=-1  DataType=auto
      settings: SignalType=auto
  Alpha sensor (with initial state) : simulink_extras/Additional Linear/Transfer Fcn (with initial states)  N=[1]  D="[0.02  1]"  X0=x0(23)
  Altitude sensor (with initial state) : simulink_extras/Additional Linear/Transfer Fcn (with initial states)  N=[1]  D="[0.02  1]"  X0=x0(35)
  Beta sensor (with initial state) : simulink_extras/Additional Linear/Transfer Fcn (with initial states)  N=[1]  D="[0.02  1]"  X0=x0(24)
  Demux : Demux  Outputs=28
  Mux : Mux  Inputs=28
      settings: DisplayOption=none
  Nz sensor (with initial state) : simulink_extras/Additional Linear/Transfer Fcn (with initial states)  N=[0.0001903 0.005346 1]  D=[0.0004942 0.03082 1]  X0=[x0(36) x0(37)]
  Pb sensor (with initial state) : simulink_extras/Additional Linear/Transfer Fcn (with initial states)  N=[0.0001903 0.005346 1]  D=[0.0004942 0.03082 1]  X0=[x0(25) x0(26)]
  Phi sensor (with initial state) : simulink_extras/Additional Linear/Transfer Fcn (with initial states)  N=[1]  D=[0.00104 0.0323 1]  X0=[x0(33) x0(34)]
  Qb sensor (with initial state) : simulink_extras/Additional Linear/Transfer Fcn (with initial states)  N=[0.0001903 0.005346 1]  D=[0.0004942 0.03082 1]  X0=[x0(27) x0(28)]
  Rb sensor (with initial state) : simulink_extras/Additional Linear/Transfer Fcn (with initial states)  N=[0.0001903 0.005346 1]  D=[0.0004942 0.03082 1]  X0=[x0(29) x0(30)]
  Subsystem To Gain-Scheduling : Subsystem
  Sum{2..3,6..7} (4 alike) : Sum  Inputs=++  SaturateOnIntegerOverflow=on
  Terminator : Terminator
  Theta sensor (with initial state) : simulink_extras/Additional Linear/Transfer Fcn (with initial states)  N=[1]  D=[0.00104 0.0323 1]  X0=[x0(31) x0(32)]
  To Workspace : ToWorkspace  VariableName=alt  SampleTime=-1  SaveFormat=Matrix
  To Workspace1 : ToWorkspace  VariableName=mach  SampleTime=-1  SaveFormat=Matrix
  Vt sensor (with initial state) : simulink_extras/Additional Linear/Transfer Fcn (with initial states)  N=[1]  D="[0.02  1]"  X0=x0(22)
  altitude2z : Gain  Gain=-1  SaturateOnIntegerOverflow=off
  dVt_err : Constant  Value=dVt_err
  dalpha_err : Constant  Value=dalpha_err
  dalt_err : Constant  Value=dalt_err
  dbeta_err : Constant  Value=dbeta_err
  z2altitude : Gain  Gain=-1  SaturateOnIntegerOverflow=off
  admire_sensed_out : Outport  Port=1
  wires:
  Demux/24 -> Mux/24
  Demux/25 -> Mux/25
  Demux/26 -> Mux/26
  Demux/27 -> Mux/27
  Demux/28 -> Mux/28
  admire_out/1 -> Demux/1
  Qb sensor (with initial state)/1 -> Mux/5
  Demux/11 -> Mux/11
  Demux/13 -> Mux/13
  Demux/14 -> Mux/14
  Demux/5 -> Qb sensor (with initial state)/1
  Demux/4 -> Pb sensor (with initial state)/1
  Pb sensor (with initial state)/1 -> Mux/4
  Alpha sensor (with initial state)/1 -> Mux/2
  Demux/6 -> Rb sensor (with initial state)/1
  Rb sensor (with initial state)/1 -> Mux/6
  Demux/8 -> Theta sensor (with initial state)/1
  Theta sensor (with initial state)/1 -> Mux/8
  Demux/15 -> Mux/15
  Demux/16 -> Mux/16
  Demux/17 -> Mux/17
  Demux/18 -> Mux/18
  Demux/20 -> Mux/20
  Demux/22 -> Mux/22
  Demux/23 -> Mux/23
  Demux/21 -> Terminator/1
  dalpha_err/1 -> Sum3/2
  Demux/2 -> Sum3/1
  Sum3/1 -> Alpha sensor (with initial state)/1
  dbeta_err/1 -> Sum2/2
  Demux/3 -> Sum2/1
  Mux/1 -> admire_sensed_out/1
  Sum7/1 -> Vt sensor (with initial state)/1
  dVt_err/1 -> Sum7/2
  Demux/1 -> Sum7/1
  Vt sensor (with initial state)/1 -> Mux/1, Subsystem To Gain-Scheduling/1(Vt [m/s])
  Demux/9 -> Phi sensor (with initial state)/1
  Phi sensor (with initial state)/1 -> Mux/9
  Demux/7 -> Mux/7
  dalt_err/1 -> Sum6/2
  Sum6/1 -> Altitude sensor (with initial state)/1
  Demux/12 -> z2altitude/1
  z2altitude/1 -> Sum6/1
  Nz sensor (with initial state)/1 -> Mux/19
  Sum2/1 -> Beta sensor (with initial state)/1
  Beta sensor (with initial state)/1 -> Mux/3
  Demux/10 -> Mux/10
  Demux/19 -> Nz sensor (with initial state)/1
  altitude2z/1 -> Mux/12
  Altitude sensor (with initial state)/1 -> Subsystem To Gain-Scheduling/2(alt [m]), altitude2z/1, To Workspace/1
  Subsystem To Gain-Scheduling/1(Mach) -> Mux/21, To Workspace1/1

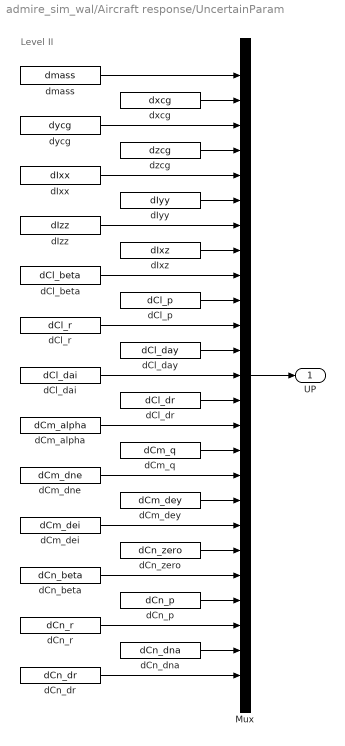
== system admire_sim_wal/Aircraft response/UncertainParam ==
  note: Level II
  Mux : Mux  Inputs=25
      settings: DisplayOption=none
  "dCl_beta " : Constant  Value=dCl_beta
  "dCl_dai " : Constant  Value=dCl_dai
  dCl_day : Constant  Value=dCl_day
  "dCl_dr " : Constant  Value=dCl_dr
  "dCl_p " : Constant  Value=dCl_p
  "dCl_r " : Constant  Value=dCl_r
  "dCm_alpha " : Constant  Value=dCm_alpha
  "dCm_dei " : Constant  Value=dCm_dei
  "dCm_dey " : Constant  Value=dCm_dey
  "dCm_dne " : Constant  Value=dCm_dne
  "dCm_q " : Constant  Value=dCm_q
  "dCn_beta " : Constant  Value=dCn_beta
  dCn_dna : Constant  Value=dCn_dna
  "dCn_dr " : Constant  Value=dCn_dr
  "dCn_p " : Constant  Value=dCn_p
  "dCn_r " : Constant  Value=dCn_r
  dCn_zero : Constant  Value=dCn_zero
  dIxx : Constant  Value=dIxx
  dIxz : Constant  Value=dIxz
  "dIyy " : Constant  Value=dIyy
  "dIzz " : Constant  Value=dIzz
  "dmass " : Constant  Value=dmass
  dxcg : Constant  Value=dxcg
  "dycg " : Constant  Value=dycg
  "dzcg " : Constant  Value=dzcg
  UP : Outport  Port=1  InitialOutput=0
  wires:
  dCn_dna/1 -> Mux/24
  "dmass "/1 -> Mux/1
  "dycg "/1 -> Mux/3
  dxcg/1 -> Mux/2
  "dzcg "/1 -> Mux/4
  dIxx/1 -> Mux/5
  "dIyy "/1 -> Mux/6
  "dIzz "/1 -> Mux/7
  dIxz/1 -> Mux/8
  "dCl_beta "/1 -> Mux/9
  "dCl_p "/1 -> Mux/10
  "dCl_r "/1 -> Mux/11
  dCl_day/1 -> Mux/12
  "dCl_dai "/1 -> Mux/13
  "dCl_dr "/1 -> Mux/14
  "dCm_alpha "/1 -> Mux/15
  "dCm_q "/1 -> Mux/16
  "dCm_dey "/1 -> Mux/18
  dCn_zero/1 -> Mux/20
  "dCn_p "/1 -> Mux/22
  Mux/1 -> UP/1
  "dCm_dne "/1 -> Mux/17
  "dCm_dei "/1 -> Mux/19
  "dCn_beta "/1 -> Mux/21
  "dCn_dr "/1 -> Mux/25
  "dCn_r "/1 -> Mux/23

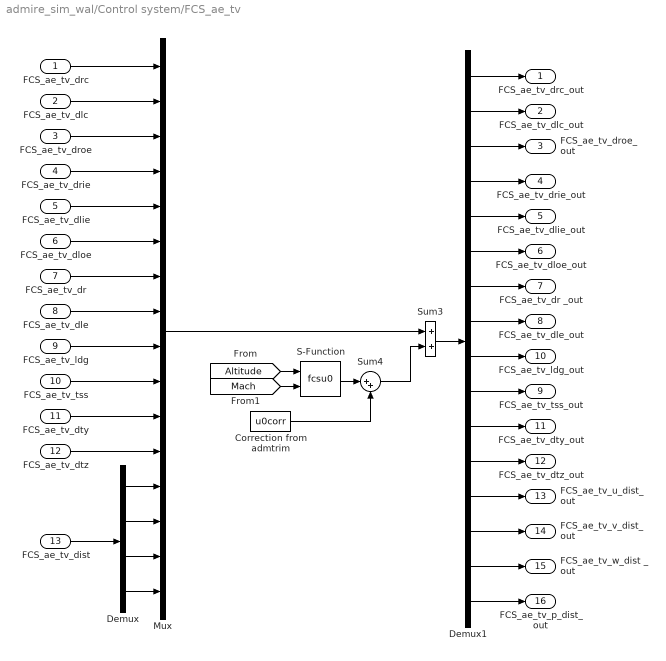
== system admire_sim_wal/Control system/FCS_ae_tv ==
  FCS_ae_tv_drc : Inport  Port=1  PortWidth=-1  SampleTime=-1  DataType=auto
      settings: SignalType=auto
  FCS_ae_tv_dlc : Inport  Port=2  PortWidth=-1  SampleTime=-1  DataType=auto
      settings: SignalType=auto
  FCS_ae_tv_droe : Inport  Port=3  PortWidth=-1  SampleTime=-1  DataType=auto
      settings: SignalType=auto
  FCS_ae_tv_drie : Inport  Port=4  PortWidth=-1  SampleTime=-1  DataType=auto
      settings: SignalType=auto
  FCS_ae_tv_dlie : Inport  Port=5  PortWidth=-1  SampleTime=-1  DataType=auto
      settings: SignalType=auto
  FCS_ae_tv_dloe : Inport  Port=6  PortWidth=-1  SampleTime=-1  DataType=auto
      settings: SignalType=auto
  FCS_ae_tv_dr : Inport  Port=7  PortWidth=-1  SampleTime=-1  DataType=auto
      settings: SignalType=auto
  FCS_ae_tv_dle : Inport  Port=8  PortWidth=-1  SampleTime=-1  DataType=auto
      settings: SignalType=auto
  FCS_ae_tv_ldg : Inport  Port=9  PortWidth=-1  SampleTime=-1  DataType=auto
      settings: SignalType=auto
  FCS_ae_tv_tss : Inport  Port=10  PortWidth=-1  SampleTime=-1  DataType=auto
      settings: SignalType=auto
  FCS_ae_tv_dty : Inport  Port=11  PortWidth=-1  SampleTime=-1  DataType=auto
      settings: SignalType=auto
  FCS_ae_tv_dtz : Inport  Port=12  PortWidth=-1  SampleTime=-1  DataType=auto
      settings: SignalType=auto
  FCS_ae_tv_dist : Inport  Port=13  PortWidth=-1  SampleTime=-1  DataType=auto
      settings: SignalType=auto
  Correction from admtrim : Constant  Value=u0corr
  Demux : Demux  Outputs=4
  Demux1 : Demux  Outputs=16
  Mux : Mux  Inputs=16
  S-Function : S-Function  FunctionName=fcsu0  PortCounts=[]  SFunctionModules=''
  Sum3 : Sum  Inputs=++  SaturateOnIntegerOverflow=on
  Sum4 : Sum  Inputs=|++  SaturateOnIntegerOverflow=on
  "FCS_ae_tv_drc_out " : Outport  Port=1
  "FCS_ae_tv_dlc_out " : Outport  Port=2
  "FCS_ae_tv_droe_out " : Outport  Port=3
  "FCS_ae_tv_drie_out " : Outport  Port=4
  "FCS_ae_tv_dlie_out " : Outport  Port=5
  "FCS_ae_tv_dloe_out " : Outport  Port=6
  FCS_ae_tv_dr _out : Outport  Port=7
  "FCS_ae_tv_dle_out " : Outport  Port=8
  "FCS_ae_tv_tss_out " : Outport  Port=9
  "FCS_ae_tv_ldg_out " : Outport  Port=10
  FCS_ae_tv_dty_out : Outport  Port=11
  "FCS_ae_tv_dtz_out " : Outport  Port=12
  "FCS_ae_tv_u_dist_out " : Outport  Port=13
  "FCS_ae_tv_v_dist_out " : Outport  Port=14
  FCS_ae_tv_w_dist _out : Outport  Port=15
  "FCS_ae_tv_p_dist_out " : Outport  Port=16
  wires:
  FCS_ae_tv_dist/1 -> Demux/1
  FCS_ae_tv_drc/1 -> Mux/1
  FCS_ae_tv_dlc/1 -> Mux/2
  FCS_ae_tv_droe/1 -> Mux/3
  FCS_ae_tv_drie/1 -> Mux/4
  FCS_ae_tv_dlie/1 -> Mux/5
  FCS_ae_tv_dloe/1 -> Mux/6
  FCS_ae_tv_dr/1 -> Mux/7
  FCS_ae_tv_dle/1 -> Mux/8
  FCS_ae_tv_dty/1 -> Mux/11
  FCS_ae_tv_dtz/1 -> Mux/12
  Demux/1 -> Mux/13
  Demux/2 -> Mux/14
  Demux/3 -> Mux/15
  Demux/4 -> Mux/16
  FCS_ae_tv_ldg/1 -> Mux/9
  FCS_ae_tv_tss/1 -> Mux/10
  Sum3/1 -> Demux1/1
  Demux1/3 -> "FCS_ae_tv_droe_out "/1
  Demux1/4 -> "FCS_ae_tv_drie_out "/1
  Demux1/5 -> "FCS_ae_tv_dlie_out "/1
  Demux1/6 -> "FCS_ae_tv_dloe_out "/1
  Demux1/7 -> FCS_ae_tv_dr _out/1
  Demux1/8 -> "FCS_ae_tv_dle_out "/1
  Demux1/11 -> FCS_ae_tv_dty_out/1
  Demux1/12 -> "FCS_ae_tv_dtz_out "/1
  Demux1/13 -> "FCS_ae_tv_u_dist_out "/1
  Demux1/14 -> "FCS_ae_tv_v_dist_out "/1
  Demux1/15 -> FCS_ae_tv_w_dist _out/1
  Demux1/16 -> "FCS_ae_tv_p_dist_out "/1
  Demux1/2 -> "FCS_ae_tv_dlc_out "/1
  Demux1/1 -> "FCS_ae_tv_drc_out "/1
  Demux1/9 -> "FCS_ae_tv_ldg_out "/1
  Demux1/10 -> "FCS_ae_tv_tss_out "/1
  Sum4/1 -> Sum3/2
  Mux/1 -> Sum3/1
  [Altitude] -> S-Function/1
  [Mach] -> S-Function/2
  S-Function/1 -> Sum4/1
  Correction from admtrim/1 -> Sum4/2

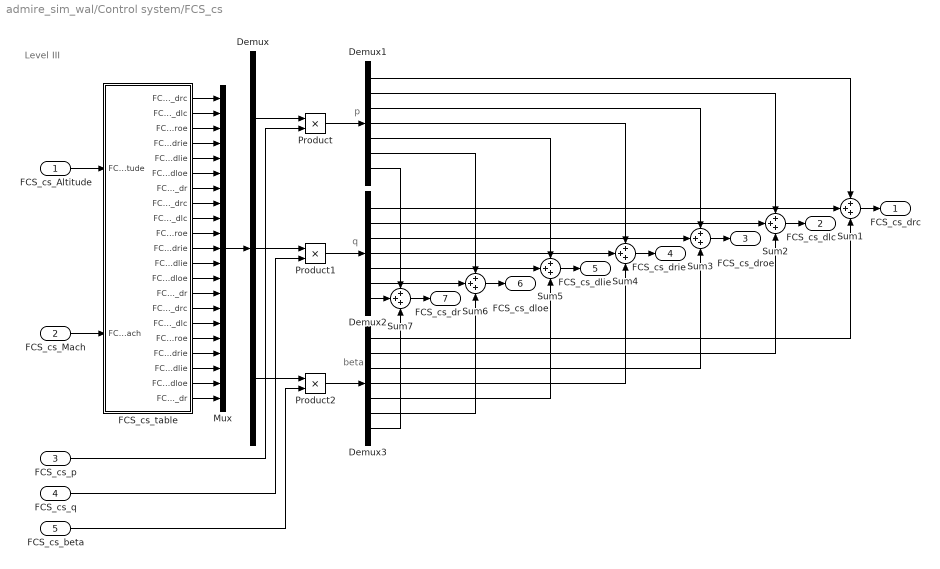
== system admire_sim_wal/Control system/FCS_cs  ==
  note: p
  note: q
  note: beta
  note: Level III
  FCS_cs_Altitude : Inport  Port=1  PortWidth=-1  SampleTime=-1  DataType=auto
      settings: SignalType=auto
  FCS_cs_Mach : Inport  Port=2  PortWidth=-1  SampleTime=-1  DataType=auto
      settings: SignalType=auto
  FCS_cs_p : Inport  Port=3  PortWidth=-1  SampleTime=-1  DataType=auto
      settings: SignalType=auto
  FCS_cs_q : Inport  Port=4  PortWidth=-1  SampleTime=-1  DataType=auto
      settings: SignalType=auto
  FCS_cs_beta : Inport  Port=5  PortWidth=-1  SampleTime=-1  DataType=auto
      settings: SignalType=auto
  Demux : Demux  Outputs=[7 7 7]
  Demux1 : Demux  Outputs=7
  Demux2 : Demux  Outputs=7
  Demux3 : Demux  Outputs=7
  FCS_cs_table : Subsystem
      mask Display: disp('FCS_cs_table')
  Mux : Mux  Inputs=21
  Product : Product  Inputs=2  SaturateOnIntegerOverflow=on
  Product1 : Product  Inputs=2  SaturateOnIntegerOverflow=on
  Product2 : Product  Inputs=2  SaturateOnIntegerOverflow=on
  Sum{1..7} (7 alike) : Sum  Inputs=3  SaturateOnIntegerOverflow=on
  FCS_cs_drc : Outport  Port=1
  FCS_cs_dlc : Outport  Port=2
  FCS_cs_droe : Outport  Port=3
  FCS_cs_drie : Outport  Port=4
  FCS_cs_dlie : Outport  Port=5
  FCS_cs_dloe : Outport  Port=6
  FCS_cs_dr : Outport  Port=7
  wires:
  Mux/1 -> Demux/1
  Demux/1 -> Product/1
  Demux/2 -> Product1/1
  Demux/3 -> Product2/1
  FCS_cs_p/1 -> Product/2
  FCS_cs_q/1 -> Product1/2
  FCS_cs_beta/1 -> Product2/2
  FCS_cs_Altitude/1 -> FCS_cs_table/1(FCS_cs_table_Altitude)
  FCS_cs_Mach/1 -> FCS_cs_table/2(FCS_cs_table_Mach)
  FCS_cs_table/1(FCS_cs_table_p_drc) -> Mux/1
  FCS_cs_table/2(FCS_cs_table_p_dlc) -> Mux/2
  FCS_cs_table/3(FCS_cs_table_p_droe) -> Mux/3
  FCS_cs_table/4(FCS_cs_table_p_drie) -> Mux/4
  FCS_cs_table/5(FCS_cs_table_p_dlie) -> Mux/5
  FCS_cs_table/6(FCS_cs_table_p_dloe) -> Mux/6
  FCS_cs_table/7(FCS_cs_table_p_dr) -> Mux/7
  FCS_cs_table/8(FCS_cs_table_q_drc) -> Mux/8
  FCS_cs_table/9(FCS_cs_table_q_dlc) -> Mux/9
  FCS_cs_table/10(FCS_cs_table_q_droe) -> Mux/10
  FCS_cs_table/11(FCS_cs_table_q_drie) -> Mux/11
  FCS_cs_table/12(FCS_cs_table_q_dlie) -> Mux/12
  FCS_cs_table/14(FCS_cs_table_q_dr) -> Mux/14
  FCS_cs_table/13(FCS_cs_table_q_dloe) -> Mux/13
  FCS_cs_table/15(FCS_cs_table_beta_drc) -> Mux/15
  FCS_cs_table/16(FCS_cs_table_beta_dlc) -> Mux/16
  FCS_cs_table/17(FCS_cs_table_beta_droe) -> Mux/17
  FCS_cs_table/18(FCS_cs_table_beta_drie) -> Mux/18
  FCS_cs_table/19(FCS_cs_table_beta_dlie) -> Mux/19
  FCS_cs_table/20(FCS_cs_table_beta_dloe) -> Mux/20
  FCS_cs_table/21(FCS_cs_table_beta_dr) -> Mux/21
  Product/1 -> Demux1/1
  Product1/1 -> Demux2/1
  Product2/1 -> Demux3/1
  Demux2/6 -> Sum6/2
  Demux2/7 -> Sum7/2
  Demux1/7 -> Sum7/1
  Demux3/7 -> Sum7/3
  Sum7/1 -> FCS_cs_dr/1
  Demux2/5 -> Sum5/2
  Demux1/6 -> Sum6/1
  Demux3/6 -> Sum6/3
  Sum6/1 -> FCS_cs_dloe/1
  Demux2/4 -> Sum4/2
  Demux1/5 -> Sum5/1
  Demux3/5 -> Sum5/3
  Sum5/1 -> FCS_cs_dlie/1
  Demux2/3 -> Sum3/2
  Demux1/4 -> Sum4/1
  Demux3/4 -> Sum4/3
  Sum4/1 -> FCS_cs_drie/1
  Demux2/2 -> Sum2/2
  Demux1/3 -> Sum3/1
  Demux3/3 -> Sum3/3
  Sum3/1 -> FCS_cs_droe/1
  Demux2/1 -> Sum1/2
  Demux1/2 -> Sum2/1
  Demux3/2 -> Sum2/3
  Sum2/1 -> FCS_cs_dlc/1
  Demux1/1 -> Sum1/1
  Demux3/1 -> Sum1/3
  Sum1/1 -> FCS_cs_drc/1

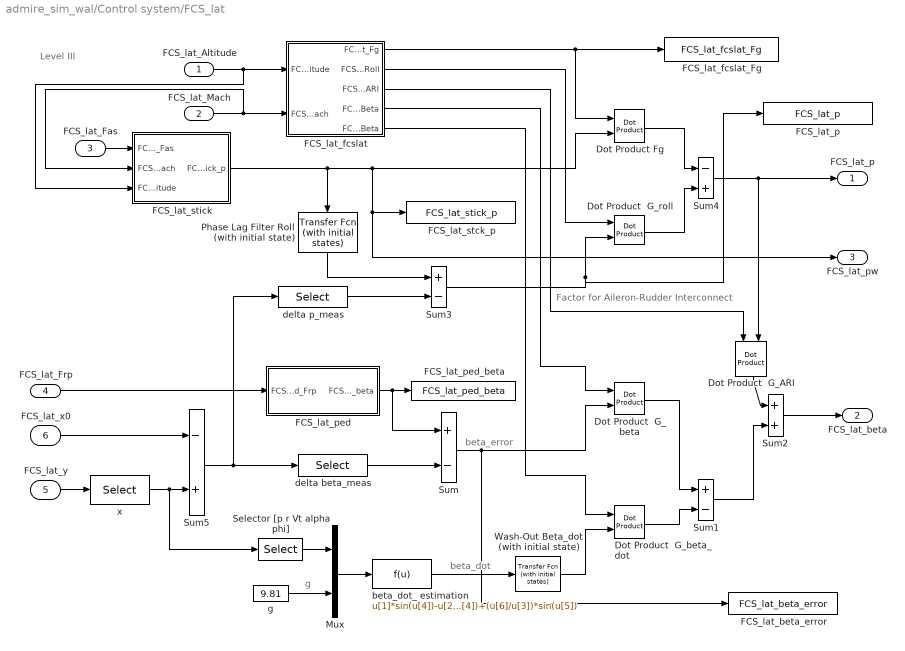
== system admire_sim_wal/Control system/FCS_lat ==
  note: g
  note: beta_dot
  note: beta_error
  note: Level III
  note: Factor for Aileron-Rudder
      | Interconnect
  "FCS_lat_Altitude " : Inport  Port=1  PortWidth=-1  SampleTime=-1  DataType=auto
      settings: SignalType=auto
  "FCS_lat_Mach " : Inport  Port=2  PortWidth=-1  SampleTime=-1  DataType=auto
      settings: SignalType=auto
  FCS_lat_Fas : Inport  Port=3  PortWidth=-1  SampleTime=-1  DataType=auto
      settings: SignalType=auto
  FCS_lat_Frp : Inport  Port=4  PortWidth=-1  SampleTime=-1  DataType=auto
      settings: SignalType=auto
  "FCS_lat_y " : Inport  Port=5  PortWidth=-1  SampleTime=-1  DataType=auto
      settings: SignalType=auto
  FCS_lat_x0 : Inport  Port=6  PortWidth=-1  SampleTime=-1  DataType=auto
      settings: SignalType=auto
  "  x" : Selector  Elements=[1:12]  InputPortWidth=28
  Dot Product Fg : simulink3/Math/Dot Product
  Dot Product  G_ARI : simulink3/Math/Dot Product  Orientation=down
  Dot Product  G_beta : simulink3/Math/Dot Product
  Dot Product  G_beta_dot : simulink3/Math/Dot Product
  Dot Product  G_roll : simulink3/Math/Dot Product
  FCS_lat_beta_error : ToWorkspace  VariableName=FCS_lat_beta_error  SampleTime=-1  SaveFormat=Matrix
  FCS_lat_fcslat : Subsystem
      mask Display: disp('Calc of lateral\namplfication\n factors')
  FCS_lat_fcslat_Fg : ToWorkspace  VariableName=FCS_lat_fcslat_Fg  SampleTime=-1  SaveFormat=Matrix
  FCS_lat_p : ToWorkspace  VariableName=FCS_lat_p  SampleTime=-1  SaveFormat=Matrix
  FCS_lat_ped : Subsystem
      mask Display: disp('FCS lateral pedal\nforce N to beta rad')
  FCS_lat_ped_beta : ToWorkspace  VariableName=FCS_lat_ped_beta  SampleTime=-1  SaveFormat=Matrix
  FCS_lat_stck_p : ToWorkspace  VariableName=FCS_lat_stick_p  SampleTime=-1  SaveFormat=Matrix
  FCS_lat_stick : Subsystem
      mask Display: disp('FCS lateral stick\ngradient\n N to rad/s')
  Mux : Mux  Inputs=2
      settings: DisplayOption=none
  Phase Lag Filter Roll (with initial state) : simulink_extras/Additional Linear/Transfer Fcn (with initial states)  Orientation=down  N=[0 1]  D="[0.25  1]"  X0=x0(39)
  Selector [p r Vt alpha phi] : Selector  Elements=[4 6 1 2 9]  InputPortWidth=12
  Sum : Sum  Inputs=+-  SaturateOnIntegerOverflow=on
  Sum1 : Sum  Inputs=+-  SaturateOnIntegerOverflow=on
  Sum2 : Sum  Inputs=++  SaturateOnIntegerOverflow=on
  Sum3 : Sum  Inputs=+-  SaturateOnIntegerOverflow=on
  Sum4 : Sum  Inputs=-+  SaturateOnIntegerOverflow=on
  Sum5 : Sum  Inputs=-+  SaturateOnIntegerOverflow=on
  Wash-Out Beta_dot (with initial state) : simulink_extras/Additional Linear/Transfer Fcn (with initial states)  N=[5 0]  D="[5  1]"  X0=x0(40)
  beta_dot_ estimation : Fcn  Expr=u[1]*sin(u[4])-u[2]*cos(u[4])+(u[6]/u[3])*sin(u[5])
  delta beta_meas : Selector  Elements=3  InputPortWidth=12
  delta p_meas : Selector  Elements=4  InputPortWidth=12
  g : Constant  Value=9.81
  "FCS_lat_p " : Outport  Port=1  InitialOutput=0
  "FCS_lat_beta " : Outport  Port=2  InitialOutput=0
  FCS_lat_pw : Outport  Port=3  InitialOutput=0
  wires:
  FCS_lat_Fas/1 -> FCS_lat_stick/1("FCS_lat_stick_Fas ")
  Phase Lag Filter Roll (with initial state)/1 -> Sum3/1
  delta p_meas/1 -> Sum3/2
  Mux/1 -> beta_dot_ estimation/1
  Selector [p r Vt alpha phi]/1 -> Mux/1
  g/1 -> Mux/2
  beta_dot_ estimation/1 -> Wash-Out Beta_dot (with initial state)/1
  Dot Product  G_roll/1 -> Sum4/2
  Dot Product Fg/1 -> Sum4/1
  Wash-Out Beta_dot (with initial state)/1 -> Dot Product  G_beta_dot/2
  Dot Product  G_beta/1 -> Sum1/1
  Dot Product  G_beta_dot/1 -> Sum1/2
  Dot Product  G_ARI/1 -> Sum2/1
  Sum2/1 -> "FCS_lat_beta "/1
  Sum1/1 -> Sum2/2
  FCS_lat_stick/1(FCS_lat_stick_p) -> Phase Lag Filter Roll (with initial state)/1, Dot Product Fg/2, FCS_lat_pw/1, FCS_lat_stck_p/1
  FCS_lat_fcslat/2(FCS_lat_fcslat_GRoll) -> Dot Product  G_roll/1
  FCS_lat_fcslat/3(FCS_lat_fcslat_GARI) -> Dot Product  G_ARI/1
  FCS_lat_fcslat/4(FCS_lat_fcslat_GBeta) -> Dot Product  G_beta/1
  FCS_lat_fcslat/5(FCS_lat_fcslat_dGBeta) -> Dot Product  G_beta_dot/1
  delta beta_meas/1 -> Sum/2
  FCS_lat_Frp/1 -> FCS_lat_ped/1(FCS_lat_ped_Frp)
  "FCS_lat_Altitude "/1 -> FCS_lat_fcslat/1(FCS_lat_fcslat_Altitude), FCS_lat_stick/3("FCS_lat_stick_Altitude ")
  "FCS_lat_Mach "/1 -> FCS_lat_stick/2("FCS_lat_stick_Mach "), FCS_lat_fcslat/2(FCS_lat_fcslat_Mach)
  "FCS_lat_y "/1 -> "  x"/1
  FCS_lat_x0/1 -> Sum5/1
  "  x"/1 -> Sum5/2, Selector [p r Vt alpha phi]/1
  Sum5/1 -> delta beta_meas/1, delta p_meas/1
  FCS_lat_fcslat/1(FCS_lat_fcslat_Fg) -> Dot Product Fg/1, FCS_lat_fcslat_Fg/1
  FCS_lat_ped/1(FCS_lat_ped_beta) -> FCS_lat_ped_beta/1, Sum/1
  Sum/1 -> Dot Product  G_beta/2, FCS_lat_beta_error/1
  Sum4/1 -> Dot Product  G_ARI/2, "FCS_lat_p "/1
  Sum3/1 -> Dot Product  G_roll/2, FCS_lat_p/1
